simulink model "sampleModel105"  (R2021b)
settings: Solver=VariableStepAuto  StartTime=0.0  StopTime=10.0  RelTol=1e-3
undefined symbols (not defined in the file or in its folder): DiscIntNeverNeededParam, magnitude, Newton, Raphson
libraries: simulink x4, slpidlib x1
settings Model: Creator=user  LastModifiedBy=user

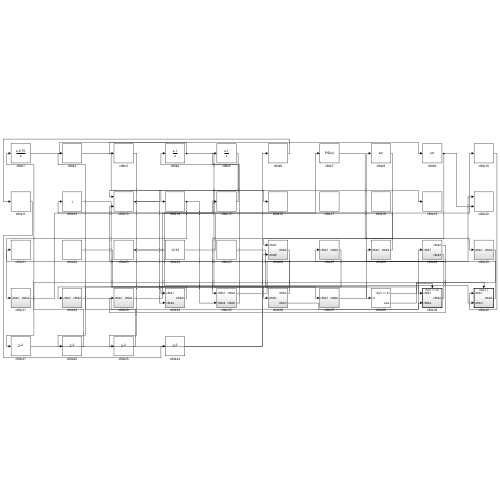
[thumbnail: Simulink's stored preview of the top-level diagram]
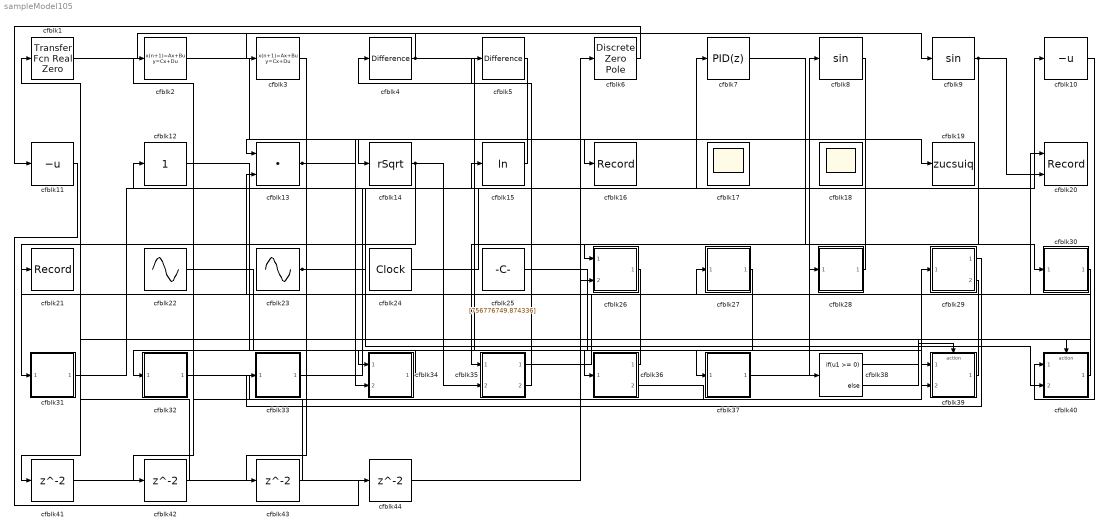
== system sampleModel105 ==
  cfblk1 : simulink/Discrete/Transfer Fcn Real Zero  ZeroZ=0.75  ICPrevInput=0.0  DoSatur=off
      settings: SourceProductBaseCode=SL
  cfblk10 : UnaryMinus
  cfblk11 : UnaryMinus
  cfblk12 : simulink/Math Operations/Slider Gain  gain=1  low=0  high=2
  cfblk13 : DotProduct  InputSameDT=on  OutDataTypeStr=Inherit: Inherit via internal rule
  cfblk14 : Sqrt  Operator=rSqrt  AlgorithmType=Newton-Raphson  SaturateOnIntegerOverflow=on
  cfblk15 : Math  Operator=log  SaturateOnIntegerOverflow=on
  cfblk16 : Record  FileSettingsInternal="{\"entries\":[{\"content\":{\"excelSettings\":{\"content\":{},\"type\":\"Streamout.ExcelSettings\"}},\"type\":\"Streamout.FileSettingStorage\",\"uuid\":\"ddb8cd18-c12f-4860-9dfc-a54a25d37713\"}],\"packageUris\":[\"http://schema.mathworks.com/mf0/streamout_blocks/R2020a\"],\"version\":\"1.0\"}"  SignalsInternal="{\"entries\":[{\"content\":{\"signals\":[{\"content\":{\"blockPath\":[\"sampleModel105/cfblk16\"],\"channel\":[],\"dimensions\":[1],\"domain\":\"sampleModel105/cfblk16\",\"lineColor\":\"#139fff\",\"plots\":[1],\"port\":1,\"sid\":[\"\"],\"signalID\":3763,\"signalName\":\"cfblk31\"},\"type\":\"RecordBlkView.Signal\",\"uuid\":\"9e456cbc-cfe6-47fb-a5ca-52251a168298\"}]},\"type\":\"RecordBlkView.InputSignals\",\"uuid\":\"aff188d9-79ce-495a-83b5-9f3deef2797b\"}],\"packageUris\":[\"http://schema.mathworks.com/mf0/streamout_blocks/R2020a\"],\"version\":\"1.0\"}"  VisualizationBindings="{\"sparklinesplugin\":{\"info\":[{\"bindingParametersList\":[],\"subplotID\":1}]}}"
  cfblk17 : Scope
      settings: Floating=on
  cfblk18 : Scope
      settings: Floating=on
  cfblk19 : ToWorkspace  VariableName=zucsuiq  SaveFormat=Timeseries  SampleTime=-1
  cfblk2 : DiscreteStateSpace
  cfblk20 : Record  FileSettingsInternal="{\"entries\":[{\"content\":{\"excelSettings\":{\"content\":{},\"type\":\"Streamout.ExcelSettings\"}},\"type\":\"Streamout.FileSettingStorage\",\"uuid\":\"994706bd-350c-4b66-ae42-702c58b05930\"}],\"packageUris\":[\"http://schema.mathworks.com/mf0/streamout_blocks/R2020a\"],\"version\":\"1.0\"}"  Layout=[1 1]  SignalsInternal="{\"entries\":[{\"content\":{\"signals\":[{\"content\":{\"blockPath\":[\"sampleModel105/cfblk20\"],\"channel\":[],\"dimensions\":[1],\"domain\":\"sampleModel105/cfblk20\",\"lineColor\":\"#a2142f\",\"plots\":[1],\"port\":1,\"sid\":[\"\"],\"signalID\":3767,\"signalName\":\"cfblk35:1\"},\"type\":\"RecordBlkView.Signal\",\"uuid\":\"5d14dbdc-6690-4294-8c36-7d91aadc88e1\"},{\"content\":{\"blockPath\":[\"sampleModel105/cfblk20\"],\"channel\":[],\"dimensions\":[1],\"domain\":\"sampleModel105/cfblk20\",\"lineColor\":\"#139fff\",\"plots\":[1],\"port\":2,\"sid\":[\"\"],\"signalID\":3771,\"signalName\":\"cfblk9\"},\"type\":\"RecordBlkView.Signal\",\"uuid\":\"fa119035-5c6e-4293-ac48-37ef39e509bf\"}]},\"type\":\"RecordBlkView.InputSignals\",\"uuid\":\"f9f6f185-69b6-43c0-9efd-025b92a68dbe\"}],\"packageUris\":[\"http://schema.mathworks.com/mf0/streamout_blocks/R2020a\"],\"version\":\"1.0\"}"  VisualizationBindings="{\"xyplotplugin\":{\"info\":[{\"series\":[{\"bindingParametersList\":[{\"parameter\":\"X-Axis\",\"signalID\":3767,\"signalName\":\"cfblk35:1\"},{\"parameter\":\"Y-Axis\",\"signalID\":3771,\"signalName\":\"cfblk9\"}],\"seriesID\":40349}],\"subplotID\":1}]}}"  CompatibilityTag=XY
  cfblk21 : Record  FileSettingsInternal="{\"entries\":[{\"content\":{\"excelSettings\":{\"content\":{},\"type\":\"Streamout.ExcelSettings\"}},\"type\":\"Streamout.FileSettingStorage\",\"uuid\":\"5933467f-9b3e-48b0-a70a-d69cf6b792e4\"}],\"packageUris\":[\"http://schema.mathworks.com/mf0/streamout_blocks/R2020a\"],\"version\":\"1.0\"}"  SignalsInternal="{\"entries\":[{\"content\":{\"signals\":[{\"content\":{\"blockPath\":[\"sampleModel105/cfblk21\"],\"channel\":[],\"dimensions\":[1],\"domain\":\"sampleModel105/cfblk21\",\"lineColor\":\"#64d413\",\"plots\":[1],\"port\":1,\"sid\":[\"\"],\"signalID\":3775,\"signalName\":\"cfblk39\"},\"type\":\"RecordBlkView.Signal\",\"uuid\":\"a37ccbd4-b422-4b4a-b4e3-4f464335f5ed\"}]},\"type\":\"RecordBlkView.InputSignals\",\"uuid\":\"58064e48-9d8c-465b-afa7-76fbacd90a10\"}],\"packageUris\":[\"http://schema.mathworks.com/mf0/streamout_blocks/R2020a\"],\"version\":\"1.0\"}"  VisualizationBindings="{\"sparklinesplugin\":{\"info\":[{\"bindingParametersList\":[],\"subplotID\":1}]}}"
  cfblk22 : Sin  Amplitude=[-767424050.346125]  Bias=[-835202544.740925]  SampleTime=0
  cfblk23 : Sin  Amplitude=[-580302716.894803]  Bias=[-692271995.278135]  SampleTime=0
  cfblk24 : DigitalClock
  cfblk25 : Constant  Value=[756776749.874336]  SampleTime=1
  cfblk26 : Subsystem
  cfblk27 : Subsystem
  cfblk28 : Subsystem
  cfblk29 : Subsystem
  cfblk3 : DiscreteStateSpace
  cfblk30 : Subsystem
  cfblk31 : Subsystem
  cfblk32 : Subsystem
  cfblk33 : Subsystem
  cfblk34 : Subsystem
  cfblk35 : Subsystem
  cfblk36 : Subsystem
  cfblk37 : Subsystem
  cfblk38 : If  IfExpression=u1 >= 0  SampleTime=1
  cfblk39 : Subsystem  TreatAsAtomicUnit=on
  cfblk4 : simulink/Discrete/Difference  ICPrevInput=0.0  OutMin=[]  OutMax=[]  OutDataTypeStr=Inherit: Inherit via back propagation  OutDataType=fixdt(1, 16)  OutScaling=2^-10  DoSatur=off
  cfblk40 : Subsystem  TreatAsAtomicUnit=on
  cfblk{41..44} (4 alike) : Delay  SampleTime=1
  cfblk5 : simulink/Discrete/Difference  ICPrevInput=0.0  OutMin=[]  OutMax=[]  OutDataTypeStr=Inherit: Inherit via back propagation  OutDataType=fixdt(1, 16)  OutScaling=2^-10  DoSatur=off
  cfblk6 : DiscreteZeroPole  Poles=[0 0.5]  Gain=1
  cfblk7 : slpidlib/PID Controller  Controller=PID  Form=Parallel  TimeDomain=Discrete-time  UseExternalTs=off  SampleTime=1  IntegratorMethod=Forward Euler  FilterMethod=Forward Euler  ControllerParametersSource=internal  P=1  I=1  D=0  UseFilter=on  N=100  TunerSelectOption=Transfer Function Based (PID Tuner App)  InitialConditionSource=internal  InitialConditionForIntegrator=0  InitialConditionForFilter=0  DifferentiatorICPrevScaledInput=0  ExternalReset=none  TrackingMode=off  Kt=1  LimitOutput=off  SatLimitsSource=internal  UpperSaturationLimit=inf  LowerSaturationLimit=-inf  LinearizeAsGain=off  AntiWindupMode=none  Kb=1  POutMin=[]  POutMax=[]  IOutMin=[]  IOutMax=[]  DOutMin=[]  DOutMax=[]  NOutMin=[]  NOutMax=[]  SumOutMin=[]  SumOutMax=[]  SaturationOutMin=[]  SaturationOutMax=[]  PParamMin=[]  PParamMax=[]  IParamMin=[]  IParamMax=[]  DParamMin=[]  DParamMax=[]  NParamMin=[]  NParamMax=[]  KbParamMin=[]  KbParamMax=[]  KtParamMin=[]  KtParamMax=[]  KbOutMin=[]  KbOutMax=[]  KtOutMin=[]  KtOutMax=[]  IntegratorOutMin=[]  IntegratorOutMax=[]  FilterOutMin=[]  FilterOutMax=[]  SumI1OutMin=[]  SumI1OutMax=[]  SumI2OutMin=[]  SumI2OutMax=[]  SumI3OutMin=[]  SumI3OutMax=[]  SumI4OutMin=[]  SumI4OutMax=[]  SumDOutMin=[]  SumDOutMax=[]  DifferentiatorOutMin=[]  DifferentiatorOutMax=[]  FilterDiffOutCoefMin=[]  FilterDiffOutCoefMax=[]  ReciprocalOutMin=[]  ReciprocalOutMax=[]  SumDenOutMin=[]  SumDenOutMax=[]  SumNumOutMin=[]  SumNumOutMax=[]  DivideOutMin=[]  DivideOutMax=[]  UdiffTsProdOutMin=[]  UdiffTsProdOutMax=[]  NTsProdOutMin=[]  NTsProdOutMax=[]  UintegralTsProdOutMin=[]  UintegralTsProdOutMax=[]  UngainTsProdOutMin=[]  UngainTsProdOutMax=[]  IntegratorContinuousStateAttributes=''  IntegratorStateMustResolveToSignalObject=off  IntegratorRTWStateStorageClass=Auto  FilterContinuousStateAttributes=''  FilterStateMustResolveToSignalObject=off  FilterRTWStateStorageClass=Auto  ParallelPVariant=InternalParameters  IdealPVariant=Disabled  IVariant=InternalParameters  DVariant=InternalParameters  IntegratorVariant=Discrete  SatVariant=Disabled  AWVariant=Passthrough  PCopyVariant=Disabled  TRVariant=Disabled  FdbkBlocksVariant=Forward  IdealPFdbkVariant=Disabled  SatFdbkVariant=Disabled  DerivativeFilterVariant=ForwardEulerFilter  NVariant=InternalParameters  NCopyVariant=Disabled  FilterICVariant=InternalICsFilter  IntegratorICVariant=InternalICs  ExternalResetVariant=Disabled  TRSumVariant=Passthrough  SumFdbkVariant=Disabled  SumVariant=Sum_PID  TsampFilterVariant=InternalTs  TsampNgainVariant=Passthrough  TsampIntegralVariant=Passthrough  ExternalSaturationOutDataTypeStr=Inherit: Same as second input
  cfblk8 : Trigonometry
  cfblk9 : Trigonometry
  wires:
  cfblk24/1 -> cfblk10/1
  cfblk34/1(cfblk2) -> cfblk32/1(cfblk1)
  cfblk37/1(cfblk2) -> cfblk8/1
  cfblk2/1 -> cfblk14/1
  cfblk32/1(cfblk2) -> cfblk29/1(cfblk1)
  cfblk31/1(cfblk2) -> cfblk16/1
  cfblk25/1 -> cfblk37/1(cfblk1)
  cfblk29/1(cfblk2) -> cfblk33/1(cfblk1)
  cfblk7/1 -> cfblk30/1(cfblk1)
  cfblk6/1 -> cfblk11/1
  cfblk4/1 -> cfblk36/1(cfblk1), cfblk3/1
  cfblk33/1(cfblk2) -> cfblk7/1
  cfblk1/1 -> cfblk9/1
  cfblk15/1 -> cfblk5/1
  cfblk14/1 -> cfblk31/1(cfblk1), cfblk35/2(cfblk4)
  cfblk23/1 -> cfblk15/1, cfblk40/2(cfblk3)
  cfblk35/1(cfblk2) -> cfblk20/1
  cfblk29/2(cfblk3) -> cfblk28/1(cfblk1)
  cfblk26/1(cfblk2) -> cfblk34/1(cfblk1)
  cfblk40/1(cfblk2) -> cfblk27/1(cfblk1)
  cfblk35/2(cfblk5) -> cfblk4/1
  cfblk8/1 -> cfblk35/1(cfblk1)
  cfblk12/1 -> cfblk38/1
  cfblk13/1 -> cfblk34/2(cfblk4), cfblk19/1
  cfblk28/1(cfblk2) -> cfblk12/1
  cfblk22/1 -> cfblk39/1(cfblk1)
  cfblk9/1 -> cfblk26/1(cfblk1), cfblk20/2
  cfblk39/1(cfblk2) -> cfblk21/1
  cfblk5/1 -> cfblk13/1
  cfblk10/1 -> cfblk40/1(cfblk1)
  cfblk36/1(cfblk2) -> cfblk13/2
  cfblk36/2(cfblk3) -> cfblk39/2(cfblk4)
  cfblk38/1 -> cfblk39/Action
  cfblk38/2 -> cfblk40/Action
  cfblk30/1(cfblk2) -> cfblk41/1
  cfblk41/1 -> cfblk26/2(cfblk5)
  cfblk27/1(cfblk2) -> cfblk42/1
  cfblk42/1 -> cfblk1/1
  cfblk3/1 -> cfblk43/1
  cfblk43/1 -> cfblk2/1
  cfblk11/1 -> cfblk44/1
  cfblk44/1 -> cfblk6/1

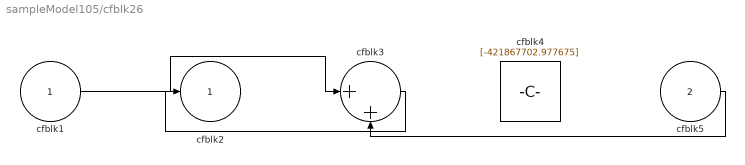
== system sampleModel105/cfblk26 ==
  cfblk1 : Inport
  cfblk5 : Inport  Port=2
  cfblk3 : Sum  Inputs=|++
  cfblk4 : Constant  Value=[-421867702.977675]  SampleTime=1
  cfblk2 : Outport
  wires:
  cfblk1/1 -> cfblk3/1
  cfblk3/1 -> cfblk2/1
  cfblk5/1 -> cfblk3/2

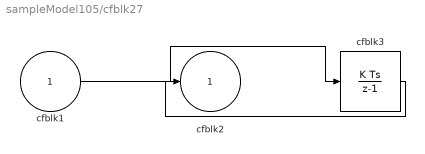
== system sampleModel105/cfblk27 ==
  cfblk1 : Inport
  cfblk3 : DiscreteIntegrator  ICPrevOutput=DiscIntNeverNeededParam  ICPrevScaledInput=DiscIntNeverNeededParam
  cfblk2 : Outport
  wires:
  cfblk1/1 -> cfblk3/1
  cfblk3/1 -> cfblk2/1

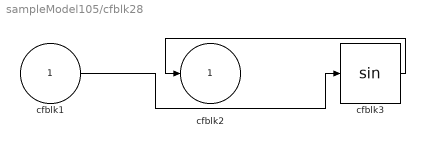
== system sampleModel105/cfblk28 ==
  cfblk1 : Inport
  cfblk3 : Trigonometry
  cfblk2 : Outport
  wires:
  cfblk3/1 -> cfblk2/1
  cfblk1/1 -> cfblk3/1

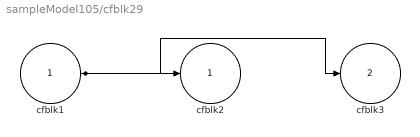
== system sampleModel105/cfblk29 ==
  cfblk1 : Inport
  cfblk2 : Outport
  cfblk3 : Outport  Port=2
  wires:
  cfblk1/1 -> cfblk2/1, cfblk3/1

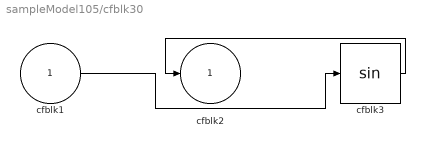
== system sampleModel105/cfblk30 ==
  cfblk1 : Inport
  cfblk3 : Trigonometry
  cfblk2 : Outport
  wires:
  cfblk3/1 -> cfblk2/1
  cfblk1/1 -> cfblk3/1

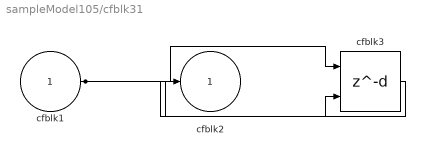
== system sampleModel105/cfblk31 ==
  cfblk1 : Inport
  cfblk3 : Delay  DelayLengthSource=Input port  SampleTime=1
      settings: InputPortMap=u0,p1
  cfblk2 : Outport
  wires:
  cfblk1/1 -> cfblk3/1, cfblk3/2
  cfblk3/1 -> cfblk2/1

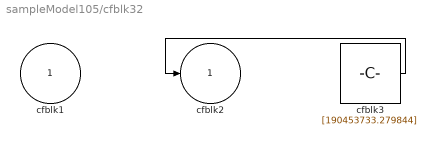
== system sampleModel105/cfblk32 ==
  cfblk1 : Inport
  cfblk3 : Constant  Value=[190453733.279844]  SampleTime=1
  cfblk2 : Outport
  wires:
  cfblk3/1 -> cfblk2/1

== system sampleModel105/cfblk33 ==
  cfblk1 : Inport
  cfblk3 : Delay  SampleTime=1
  cfblk2 : Outport
  wires:
  cfblk1/1 -> cfblk3/1
  cfblk3/1 -> cfblk2/1

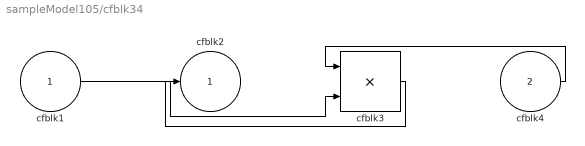
== system sampleModel105/cfblk34 ==
  cfblk1 : Inport
  cfblk4 : Inport  Port=2
  cfblk3 : Product
  cfblk2 : Outport
  wires:
  cfblk4/1 -> cfblk3/1
  cfblk1/1 -> cfblk3/2
  cfblk3/1 -> cfblk2/1

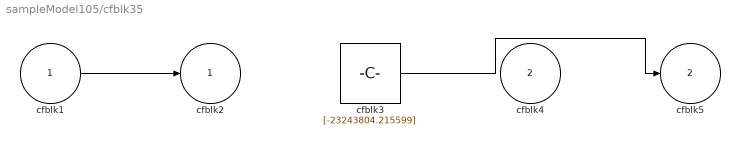
== system sampleModel105/cfblk35 ==
  cfblk1 : Inport
  cfblk4 : Inport  Port=2
  cfblk3 : Constant  Value=[-23243804.215599]  SampleTime=1
  cfblk2 : Outport
  cfblk5 : Outport  Port=2
  wires:
  cfblk3/1 -> cfblk5/1
  cfblk1/1 -> cfblk2/1

== system sampleModel105/cfblk36 ==
  cfblk1 : Inport
  cfblk2 : Outport
  cfblk3 : Outport  Port=2
  wires:
  cfblk1/1 -> cfblk2/1, cfblk3/1

== system sampleModel105/cfblk37 ==
  cfblk1 : Inport
  cfblk3 : Math  Operator=magnitude^2  SaturateOnIntegerOverflow=on
  cfblk2 : Outport
  wires:
  cfblk1/1 -> cfblk3/1
  cfblk3/1 -> cfblk2/1

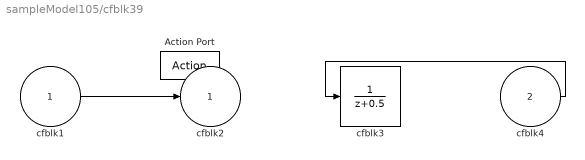
== system sampleModel105/cfblk39 ==
  cfblk1 : Inport
  cfblk4 : Inport  Port=2
  Action Port : ActionPort  ActionPortLabel=if(u1 >= 0)
  cfblk3 : DiscreteTransferFcn
  cfblk2 : Outport
  wires:
  cfblk1/1 -> cfblk2/1
  cfblk4/1 -> cfblk3/1

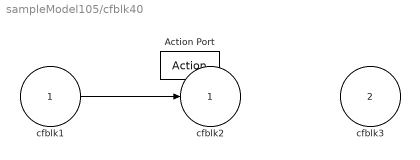
== system sampleModel105/cfblk40 ==
  cfblk1 : Inport
  cfblk3 : Inport  Port=2
  Action Port : ActionPort  ActionPortLabel=else
  cfblk2 : Outport
  wires:
  cfblk1/1 -> cfblk2/1
